simulink model "lab2_2"  (R2015b)
settings: Solver=FixedStepDiscrete  StartTime=0.0  StopTime=inf  FixedStep=0.05  RelTol=1e-3
libraries: MinSegLibrary_M2V3 x1, arduinolib x1
settings Model: SimulationMode=external  ExtModeTrigDuration=2  Creator=kando  LastModifiedBy=kando
settings OptimizationCC: OptimizeModelRefInitCode=on  LifeSpan=1  MaxStackSize=64
settings HardwareCC: ProdBitPerInt=16  ProdBitPerPointer=16  ProdLargestAtomicFloat=None  ProdWordSize=8  ProdHWDeviceType=Atmel->AVR
settings RTWCC: SystemTargetFile=ert.tlc  TemplateMakefile=ert_default_tmf  Description=Embedded Coder  Toolchain=Arduino AVR v1.6.1  BuildConfiguration=Faster Runs
settings CodeAppCC: IgnoreCustomStorageClasses=off
settings ERTTargetCC: SupportContinuousTime=on  SupportVariableSizeSignals=on

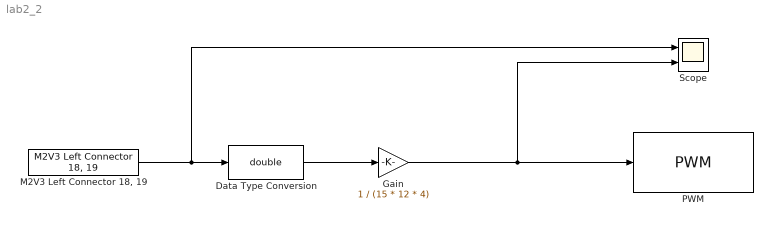
== system lab2_2 ==
  Data Type Conversion : DataTypeConversion  OutDataTypeStr=double
  Gain : Gain  Gain=1 / (15 * 12 * 4)
      settings: AttributesFormatString=|
      | k.d2a (encoder):
      | %<Gain>
  "M2V3 Left Connector 18, 19" : MinSegLibrary_M2V3/M2V3 Left Connector 18, 19  Encoder=1  PinA=19  PinB=18  PWMFSelect=3  PWMTimer=-1
  PWM : arduinolib/PWM  pinNumber=13  blockPlatform=arduino
  Scope : Scope  NumInputPorts=2
  wires:
  Data Type Conversion/1 -> Gain/1
  "M2V3 Left Connector 18, 19"/1 -> Scope/1, Data Type Conversion/1
  Gain/1 -> Scope/2, PWM/1
